simulink model "b_and_b"  (R2018b)
settings: Solver=VariableStepAuto  StartTime=0.0  StopTime=20  RelTol=1e-3
settings Model: Creator=EMiR  LastModifiedBy=EMiR

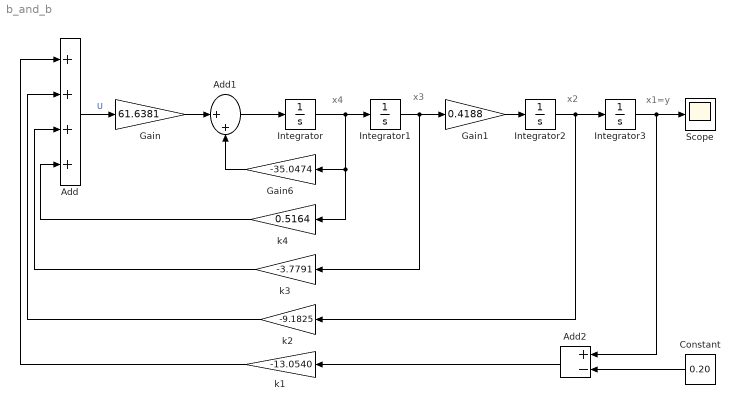
== system b_and_b ==
  note: x2
  note: x3
  note: x4
  note: x1=y
  Add : Sum  Inputs=++++
  Add1 : Sum  Inputs=|++
  Add2 : Sum  Inputs=+-
  Constant : Constant  Value=0.20
  Gain : Gain  Gain=61.6381
  Gain1 : Gain  Gain=0.4188
  Gain6 : Gain  Gain=-35.0474
  Integrator{,1..3} (4 alike) : Integrator
  Scope : Scope
  k1 : Gain  Gain=-13.0540
  k2 : Gain  Gain=-9.1825
  k3 : Gain  Gain=-3.7791
  k4 : Gain  Gain=0.5164
  wires:
  Gain/1 -> Add1/1
  Add/1 -> Gain/1  "U"
  Add1/1 -> Integrator/1
  Integrator/1 -> k4/1, Gain6/1, Integrator1/1
  Integrator1/1 -> k3/1, Gain1/1
  Gain1/1 -> Integrator2/1
  Integrator2/1 -> k2/1, Integrator3/1
  Integrator3/1 -> Add2/1, Scope/1
  Gain6/1 -> Add1/2
  k4/1 -> Add/4
  k3/1 -> Add/3
  k2/1 -> Add/2
  k1/1 -> Add/1
  Add2/1 -> k1/1
  Constant/1 -> Add2/2
